simulink model "LQR_PI_Sim"  (R2018b)
settings: Solver=FixedStepAuto  StartTime=0.0  StopTime=10  RelTol=1e-3
InitFcn:
  | LQR_ServoAeroMiahV0
values from neighbouring files (symbols this model uses):
  K = K_hat(1:m,1:n)    [LQG_Sim.m]    (also in LQR_PI_Sim.m; LQR_P_Sim.m = lqr(A,B,Q,R))
  Ki = -K_hat(1:m,n+1:n+p)    [LQG_Sim.m]    (also in LQR_PI_Sim.m)
undefined symbols (not defined in the file or in its folder): A, B, C
libraries: simulink_extras x2
settings Model: Creator=smiah-admin  LastModifiedBy=gjaniak

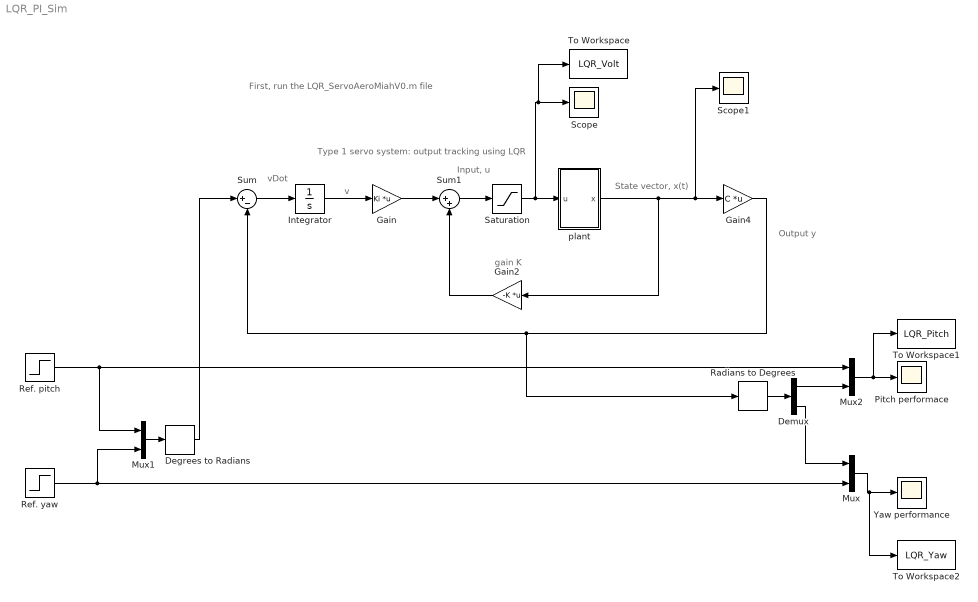
== system LQR_PI_Sim ==
  note: State vector, x(t)
  note: Input, u
  note: First, run the LQR_ServoAeroMiahV0.m file
  note: Type 1 servo system: output tracking using LQR
  note: Output y
  note: vDot
  note: gain K
  note: v
  Degrees to Radians : simulink_extras/Transformations/Degrees to Radians
  Demux : Demux  Outputs=2
  Gain : Gain  Gain=Ki  Multiplication=Matrix(K*u)
  Gain2 : Gain  Gain=-K  Multiplication=Matrix(K*u)
  Gain4 : Gain  Gain=C  Multiplication=Matrix(K*u)
  Integrator : Integrator
  Mux : Mux  Inputs=2
  Mux1 : Mux  Inputs=2
  Mux2 : Mux  Inputs=2
  Pitch performace : Scope
  Radians to Degrees : simulink_extras/Transformations/Radians to Degrees
  "Ref. pitch " : Step  Time=0  After=45  SampleTime=.01
  Ref. yaw : Step  Time=0  After=180  SampleTime=.01
  Saturation : Saturate  UpperLimit=18  LowerLimit=-18
  Scope : Scope
  Scope1 : Scope
  Sum : Sum  Inputs=|+-
  Sum1 : Sum  Inputs=|++
  To Workspace : ToWorkspace  VariableName=LQR_Volt  SaveFormat=Structure With Time  SampleTime=-1
  To Workspace1 : ToWorkspace  VariableName=LQR_Pitch  SaveFormat=Structure With Time  SampleTime=-1
  To Workspace2 : ToWorkspace  VariableName=LQR_Yaw  SaveFormat=Structure With Time  SampleTime=-1
  "Yaw performance " : Scope
  plant : Subsystem
      mask help: Plant
  wires:
  Mux/1 -> To Workspace2/1, "Yaw performance "/1
  Gain2/1 -> Sum1/2
  Gain/1 -> Sum1/1
  Sum/1 -> Integrator/1
  Integrator/1 -> Gain/1
  Gain4/1 -> Radians to Degrees/1, Sum/2
  Sum1/1 -> Saturation/1
  plant/1(x) -> Gain2/1, Scope1/1, Gain4/1
  "Ref. pitch "/1 -> Mux2/1, Mux1/1
  Ref. yaw/1 -> Mux/2, Mux1/2
  Mux1/1 -> Degrees to Radians/1
  Demux/2 -> Mux/1
  Mux2/1 -> To Workspace1/1, Pitch performace/1
  Demux/1 -> Mux2/2
  Radians to Degrees/1 -> Demux/1
  Degrees to Radians/1 -> Sum/1
  Saturation/1 -> To Workspace/1, Scope/1, plant/1(u)

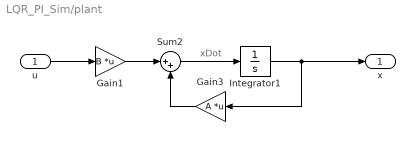
== system LQR_PI_Sim/plant ==
  note: xDot
  u : Inport
  Gain1 : Gain  Gain=B  Multiplication=Matrix(K*u)
  Gain3 : Gain  Gain=A  Multiplication=Matrix(K*u)
  Integrator1 : Integrator
  Sum2 : Sum  Inputs=|++
  x : Outport
  wires:
  Gain1/1 -> Sum2/1
  Integrator1/1 -> x/1, Gain3/1
  Gain3/1 -> Sum2/2
  Sum2/1 -> Integrator1/1
  u/1 -> Gain1/1
